simulink model "ringRoad"  (R2018b)
settings: Solver=FixedStepAuto  StartTime=0.0  StopTime=90  FixedStep=0.01  RelTol=1e-3
undefined symbols (not defined in the file or in its folder): Angular, Linear
libraries: robotlib x10, vehdynlibsteering x3, autolibshared x2, autolibutils x2, peGeneralControl x1, dspstat3 x1
settings Model: Creator=ckreienk  LastModifiedBy=ckreienk

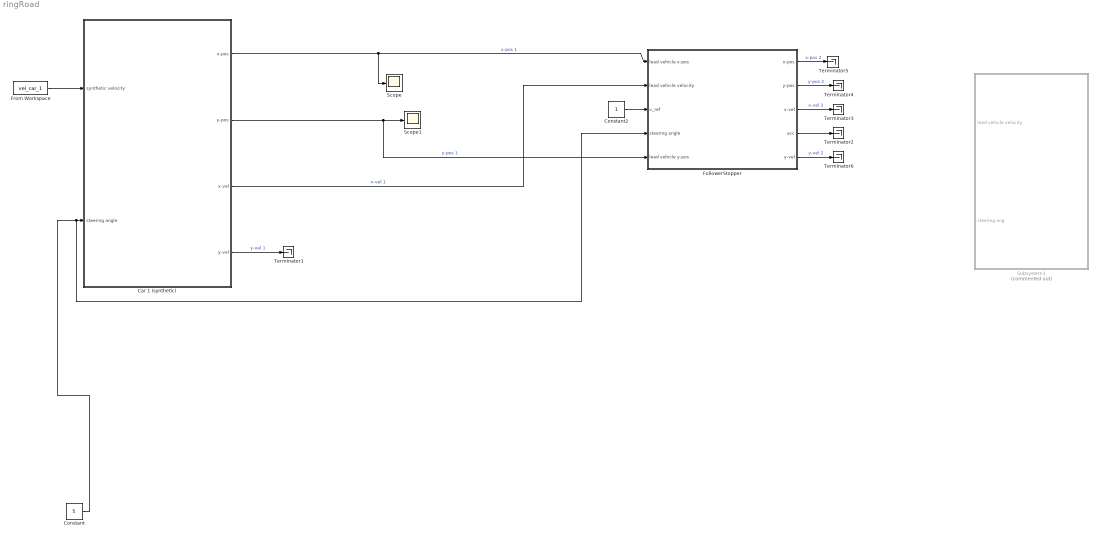
== system ringRoad ==
  Car 1 (synthetic) : Subsystem
  Constant : Constant  Value=5
  Constant2 : Constant
  FollowerStopper : Subsystem
  From Workspace : FromWorkspace  VariableName=vel_car_1
  Scope : Scope
  Scope1 : Scope
  Subsystem1 : Subsystem  Commented=on
  Terminator{1..6} (6 alike) : Terminator
  wires:
  Car 1 (synthetic)/1(x-pos) -> Scope/1, FollowerStopper/1(lead vehicle x-pos)  "x-pos 1"
  Car 1 (synthetic)/3(x-vel) -> FollowerStopper/2(lead vehicle velocity)  "x-vel 1"
  Car 1 (synthetic)/2(y-pos) -> Scope1/1, FollowerStopper/5(lead vehicle y-pos)  "y-pos 1"
  Car 1 (synthetic)/4(y-vel) -> Terminator1/1  "y-vel 1"
  Constant/1 -> FollowerStopper/4(steering angle), Car 1 (synthetic)/2(steering angle)
  From Workspace/1 -> Car 1 (synthetic)/1(synthetic velocity)
  Constant2/1 -> FollowerStopper/3(v_ref)
  FollowerStopper/4(acc) -> Terminator2/1
  FollowerStopper/3(x-vel) -> Terminator3/1  "x-vel 2"
  FollowerStopper/2(y-pos) -> Terminator4/1  "y-pos 2"
  FollowerStopper/1(x-pos) -> Terminator5/1  "x-pos 2"
  FollowerStopper/5(y-vel) -> Terminator6/1  "y-vel 2"

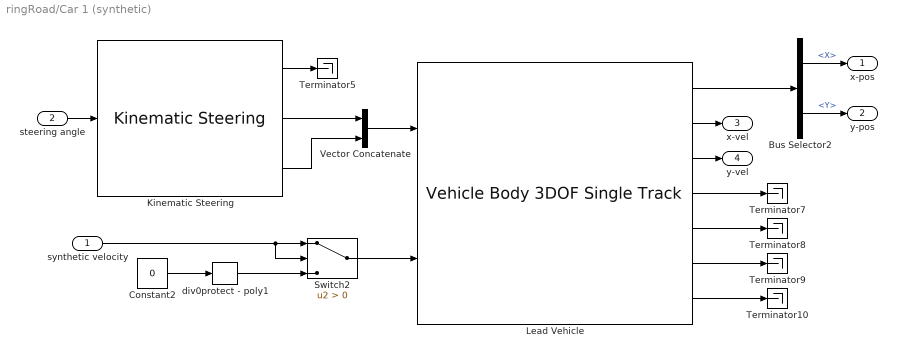
== system ringRoad/Car 1 (synthetic) ==
  synthetic velocity : Inport
  steering angle : Inport  Port=2
  Bus Selector2 : BusSelector  OutputSignals=InertFrm.Geom.Disp.X,InertFrm.Geom.Disp.Y
  Constant2 : Constant  Value=0
  Kinematic Steering : vehdynlibsteering/Kinematic Steering  StrgType=Ackerman  StrgRatioType=Constant  Loc=Front  NrmlFctr=0.01  TrckWdth=1  WhlBase=1.524  Db=0  StrgRng=1.25*pi  StrgAngBpts="[-6.2832   -5.0265   -3.7699   -2.5133   -1.2566         0    1.2566    2.5133    3.7699    5.0265    6.2832]"  StrgRatioTbl=|  StrgRatio=100  StrgArmLngth=0.1  RckCsLngth=0.5  TieRodLngth=0.248  D=0.2  PnnRadius=0.0057  PnnRadiusTbl="[0.0055    0.0055    0.0056    0.0057    0.0058    0.0057    0.0057    0.0057    0.0056    0.0055    0.0055]"  RodLngth=0.1  ParaArmLngth=0.9  aMode=2
      | [13.5000   13.3750   13.2500   13.1250   13.0000   13.0000   13.0000   13.1250   13.2500   13.3750   13.5000
      | ]
      settings: SourceProductName=Vehicle Dynamics Blockset
  Lead Vehicle : autolibshared/Vehicle Body 3DOF Single Track  trackMode=Dual  inputMode=External longitudinal velocity  frontSteerMode=on  rearSteerMode=off  windMode=off  muMode=off  extFMode=off  extMMode=off  aMode=2  NF=2  NR=2  m=2000  a=1.4  b=1.6  h=0.35  X_o=0  xdot_o=0  CalphaMode=off  sigmaMode=on  d=0  w=[1.4,1.4]  Cy_f=12e3  Cy_r=11e3  sigma_f=.1  sigma_r=.1  alpha_f_brk=[-.1 .1]  Cy_f_data=[-9e3 9e3]  alpha_r_brk=[-.1 .1]  Cy_r_data=[-9e3 9e3]  Y_o=0  ydot_o=0  Izz=4000  psi_o=0  r_o=0  Af=2  Cd=.3  Cl=.1  Cpm=.1  beta_w=[0:0.01:0.3]  Cs=[0:0.03:0.9]  Cym=[0:0.01:0.3]  Pabs=101325  Tair=273  g=9.81  mu=1  xdot_tol=.01  Fznom=5000  Fxtire_sat=7e4  Fytire_sat=7e4  longOff=0  latOff=0  vertOff=0
      settings: SourceProductName=Powertrain Blockset  SourceProductBaseCode=PW
  Switch2 : Switch  Criteria=u2 > Threshold
  Terminator{5,7..10} (5 alike) : Terminator
  Vector Concatenate : Concatenate
  div0protect - poly1 : autolibutils/div0protect - poly  thresh=1e-3  aMode=2
      settings: SourceProductName=Powertrain Blockset  SourceProductBaseCode=PW
  x-pos : Outport
  y-pos : Outport  Port=2
  x-vel : Outport  Port=3
  y-vel : Outport  Port=4
  wires:
  Lead Vehicle/6 -> Terminator9/1
  Lead Vehicle/4 -> Terminator7/1
  div0protect - poly1/1 -> Switch2/3
  Lead Vehicle/5 -> Terminator8/1
  Vector Concatenate/1 -> Lead Vehicle/1
  Lead Vehicle/7 -> Terminator10/1
  Kinematic Steering/2 -> Vector Concatenate/1
  Kinematic Steering/1 -> Terminator5/1
  synthetic velocity/1 -> Switch2/2, Switch2/1
  Switch2/1 -> Lead Vehicle/2
  Lead Vehicle/1 -> Bus Selector2/1
  Lead Vehicle/2 -> x-vel/1
  Bus Selector2/1 -> x-pos/1  "<X>"
  Bus Selector2/2 -> y-pos/1  "<Y>"
  Constant2/1 -> div0protect - poly1/1
  steering angle/1 -> Kinematic Steering/1
  Lead Vehicle/3 -> y-vel/1
  Kinematic Steering/3 -> Vector Concatenate/2

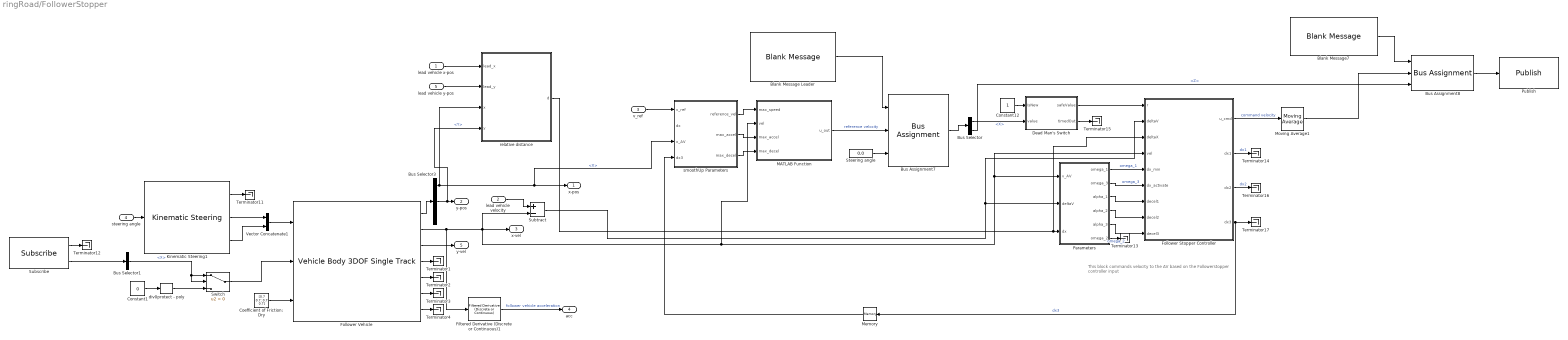
== system ringRoad/FollowerStopper ==
  note: This block commands velocity to the AV based
      | on the Followerstopper controller input
  lead vehicle x-pos : Inport
  lead vehicle velocity : Inport  Port=2
  v_ref : Inport  Port=3
  steering angle : Inport  Port=4
  lead vehicle y-pos : Inport  Port=5
  Blank Message Leader : robotlib/Blank Message  messageClass=Message  entityType=geometry_msgs/Twist  messageType=geometry_msgs/Twist  SampleTime=inf
      settings: SourceProductBaseCode=RO
  Blank Message7 : robotlib/Blank Message  messageClass=Message  entityType=geometry_msgs/Twist  messageType=geometry_msgs/Twist  SampleTime=inf
      settings: SourceProductBaseCode=RO
  Bus Assignment7 : BusAssignment  AssignedSignals=Linear.X,Angular.Z
  Bus Assignment8 : BusAssignment  AssignedSignals=Linear.X,Angular.Z
  Bus Selector : BusSelector  OutputSignals=Linear.X,Angular.Z
  Bus Selector1 : BusSelector  OutputSignals=Linear.X
  Bus Selector3 : BusSelector  OutputSignals=InertFrm.Geom.Disp.X,InertFrm.Geom.Disp.Y,InertFrm.Geom.Disp.Z
  Coefficient of Friction: Dry : Constant  Value=[0.7 0.7; 0.7 0.7]
  Constant1 : Constant  Value=0
  Constant12 : Constant
  Dead Man's Switch : Subsystem  TreatAsAtomicUnit=on  mask{stepSize=0.05, timeout=0.2}
      mask prompts: stepSize "Simulation step size"; timeout "Timeout (in seconds)"
      mask help: Interprets whether a new message has been recently received, and if so permits the data in 'value' to be passed through. Otherwise, 0 is outputted from 'safeValue'
      mask Help: Interprets whether a new message has been recently received, and if so permits the data in 'value' to be passed through. Otherwise, 0 is outputted from 'safeValue'
  Filtered Derivative (Discrete or Continuous)1 : peGeneralControl/Filtered Derivative (Discrete or Continuous)  K=1  T=0.1  B=20  A=-20  minRatio=10  Ts=-1
  Follower Stopper Controller : Subsystem
  Follower Vehicle : autolibshared/Vehicle Body 3DOF Single Track  trackMode=Dual  inputMode=External longitudinal velocity  frontSteerMode=on  rearSteerMode=off  windMode=off  muMode=on  extFMode=off  extMMode=off  aMode=2  NF=2  NR=2  m=2000  a=1.4  b=1.6  h=0.35  X_o=-5.9  xdot_o=0  CalphaMode=off  sigmaMode=on  d=0  w=[1.4,1.4]  Cy_f=12e3  Cy_r=11e3  sigma_f=.1  sigma_r=.1  alpha_f_brk=[-.1 .1]  Cy_f_data=[-9e3 9e3]  alpha_r_brk=[-.1 .1]  Cy_r_data=[-9e3 9e3]  Y_o=0.3  ydot_o=0  Izz=4000  psi_o=0  r_o=0  Af=2  Cd=.3  Cl=.1  Cpm=.1  beta_w=[0:0.01:0.3]  Cs=[0:0.03:0.9]  Cym=[0:0.01:0.3]  Pabs=101325  Tair=273  g=9.81  mu=1  xdot_tol=.01  Fznom=5000  Fxtire_sat=7e4  Fytire_sat=7e4  longOff=0  latOff=0  vertOff=0
      settings: SourceProductName=Powertrain Blockset  SourceProductBaseCode=PW
  Kinematic Steering1 : vehdynlibsteering/Kinematic Steering  StrgType=Ackerman  StrgRatioType=Constant  Loc=Front  NrmlFctr=0.01  TrckWdth=1  WhlBase=1.524  Db=0  StrgRng=1.25*pi  StrgAngBpts="[-6.2832   -5.0265   -3.7699   -2.5133   -1.2566         0    1.2566    2.5133    3.7699    5.0265    6.2832]"  StrgRatioTbl=|  StrgRatio=100  StrgArmLngth=0.1  RckCsLngth=0.5  TieRodLngth=0.248  D=0.2  PnnRadius=0.0057  PnnRadiusTbl="[0.0055    0.0055    0.0056    0.0057    0.0058    0.0057    0.0057    0.0057    0.0056    0.0055    0.0055]"  RodLngth=0.1  ParaArmLngth=0.9  aMode=2
      | [13.5000   13.3750   13.2500   13.1250   13.0000   13.0000   13.0000   13.1250   13.2500   13.3750   13.5000
      | ]
      settings: SourceProductName=Vehicle Dynamics Blockset
  MATLAB Function : MATLAB Function  TreatAsAtomicUnit=on
  Memory : Memory  InheritSampleTime=on
  Moving Average1 : dspstat3/Moving Average  Method=Sliding window  ForgettingFactorPort=off  SpecifyWindowLength=on  WindowLength=10  ForgettingFactor=0.9  SimulateUsing=Code generation
  Parameters : Subsystem
  Publish : robotlib/Publish  topicSource=Specify your own  topic=cmd_vel  messageType=geometry_msgs/Twist  messageQueueLength=1
      settings: SourceProductBaseCode=RO
  Steering angle : Constant  Value=0.0
  Subscribe : robotlib/Subscribe  topicSource=Specify your own  topic=cmd_vel  messageType=geometry_msgs/Twist  sampleTime=-1  messageQueueLength=1
      settings: SourceProductBaseCode=RO
  Subtract : Sum  Inputs=+-
  Switch : Switch  Criteria=u2 > Threshold
  Terminator{1..4,11..17} (11 alike) : Terminator
  Vector Concatenate1 : Concatenate
  div0protect - poly : autolibutils/div0protect - poly  thresh=1e-3  aMode=2
      settings: SourceProductName=Powertrain Blockset  SourceProductBaseCode=PW
  relative distance : MATLAB Function  TreatAsAtomicUnit=on
  smoothUp Parameters : Subsystem
  x-pos : Outport
  y-pos : Outport  Port=2
  x-vel : Outport  Port=3
  acc : Outport  Port=4
  y-vel : Outport  Port=5
  wires:
  Dead Man's Switch/2(timedOut) -> Terminator15/1
  Bus Selector/2 -> Bus Assignment8/3  "<Z>"
  Vector Concatenate1/1 -> Follower Vehicle/1
  Subscribe/2 -> Bus Selector1/1
  Parameters/5(alpha_3) -> Follower Stopper Controller/9(decel3)
  Parameters/3(alpha_1) -> Follower Stopper Controller/7(decel1)
  Steering angle/1 -> Bus Assignment7/3
  Follower Vehicle/3 -> y-vel/1
  Bus Selector3/1 -> x-pos/1, smoothUp Parameters/3(x_AV), relative distance/3(x)  "<X>"
  Coefficient of Friction: Dry/1 -> Follower Vehicle/3
  div0protect - poly/1 -> Switch/3
  Moving Average1/1 -> Bus Assignment8/2
  Parameters/2(omega_3) -> Follower Stopper Controller/6(dx_activate)  "omega_3"
  lead vehicle velocity/1 -> Subtract/1
  Subscribe/1 -> Terminator12/1
  Follower Vehicle/5 -> Terminator2/1
  Switch/1 -> Follower Vehicle/2
  Constant1/1 -> div0protect - poly/1
  Constant12/1 -> Dead Man's Switch/1(IsNew)
  Bus Selector3/2 -> relative distance/4(y), y-pos/1  "<Y>"
  Parameters/4(alpha_2) -> Follower Stopper Controller/8(decel2)
  Follower Vehicle/2 -> Filtered Derivative (Discrete or Continuous)1/1, Follower Stopper Controller/4(vel), Parameters/1(v_AV), MATLAB Function/2(vel), x-vel/1, Subtract/2
  Parameters/6(omega_2) -> Terminator13/1  "omega_2"
  Follower Vehicle/4 -> Terminator1/1
  Follower Stopper Controller/3(dx2) -> Terminator16/1  "dx2"
  Follower Stopper Controller/2(dx1) -> Terminator14/1  "dx1"
  Follower Vehicle/1 -> Bus Selector3/1
  Bus Selector1/1 -> Switch/1, Switch/2  "<X>"
  smoothUp Parameters/2(max_accel) -> MATLAB Function/3(max_accel)
  Blank Message Leader/1 -> Bus Assignment7/1
  Kinematic Steering1/2 -> Vector Concatenate1/1
  Dead Man's Switch/1(safeValue) -> Follower Stopper Controller/1(r)
  Bus Assignment8/1 -> Publish/1
  Follower Stopper Controller/4(dx3) -> Memory/1, Terminator17/1  "dx3"
  Kinematic Steering1/3 -> Vector Concatenate1/2
  Bus Selector/1 -> Dead Man's Switch/2(value)  "<X>"
  Follower Vehicle/7 -> Terminator4/1
  v_ref/1 -> smoothUp Parameters/1(v_ref)
  Kinematic Steering1/1 -> Terminator11/1
  smoothUp Parameters/1(reference_vel) -> MATLAB Function/1(max_speed)
  smoothUp Parameters/3(max_decel) -> MATLAB Function/4(max_decel)
  steering angle/1 -> Kinematic Steering1/1
  Bus Assignment7/1 -> Bus Selector/1
  Filtered Derivative (Discrete or Continuous)1/1 -> acc/1  "follower vehicle acceleration"
  Parameters/1(omega_1) -> Follower Stopper Controller/5(dx_min)  "omega_1"
  Follower Stopper Controller/1(u_cmd) -> Moving Average1/1  "command velocity"
  MATLAB Function/1(u_out) -> Bus Assignment7/2  "reference velocity"
  Blank Message7/1 -> Bus Assignment8/1
  Subtract/1 -> Follower Stopper Controller/2(deltaV), Parameters/2(deltaV)
  Memory/1 -> smoothUp Parameters/4(dx3)
  Follower Vehicle/6 -> Terminator3/1
  lead vehicle x-pos/1 -> relative distance/1(lead_x)
  lead vehicle y-pos/1 -> relative distance/2(lead_y)
  relative distance/1(d) -> Follower Stopper Controller/3(deltaX), Parameters/3(dx)

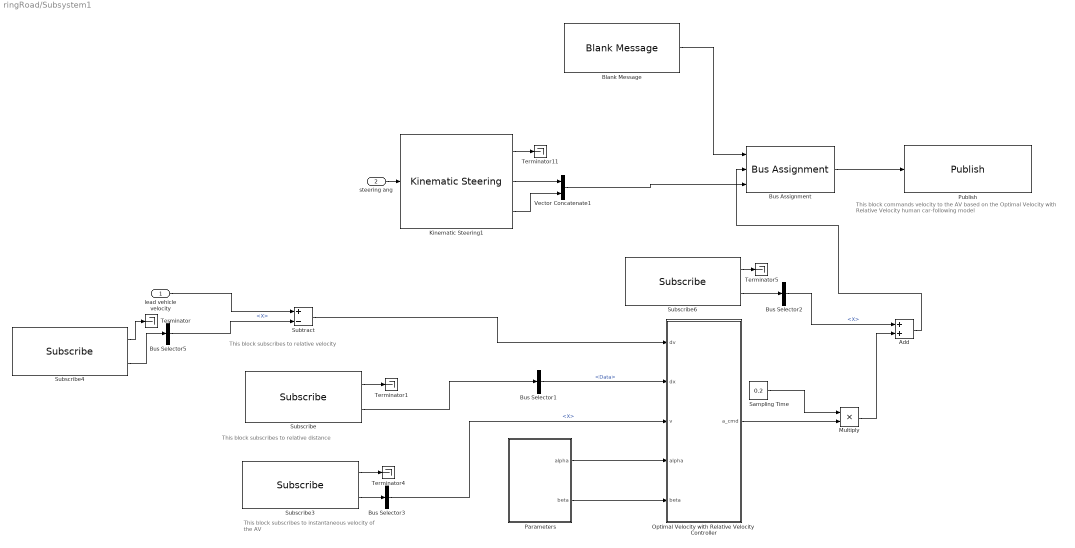
== system ringRoad/Subsystem1 ==
  note: This block subscribes to relative velocity
  note: This block subscribes to relative distance
  note: This block subscribes to
      | instantaneous velocity of the AV
  note: This block commands velocity to the AV based
      | on the Optimal Velocity with Relative Velocity
      | human car-following model
  lead vehicle velocity : Inport
  steering ang : Inport  Port=2
  Add : Sum
  Blank Message : robotlib/Blank Message  messageClass=Message  entityType=geometry_msgs/Twist  messageType=geometry_msgs/Twist  SampleTime=inf
      settings: SourceProductBaseCode=RO
  Bus Assignment : BusAssignment  AssignedSignals=Linear.X,Angular.Z
  Bus Selector1 : BusSelector  OutputSignals=Data
  Bus Selector2 : BusSelector  OutputSignals=Linear.X
  Bus Selector3 : BusSelector  OutputSignals=Linear.X
  Bus Selector5 : BusSelector  OutputSignals=Linear.X
  Kinematic Steering1 : vehdynlibsteering/Kinematic Steering  StrgType=Ackerman  StrgRatioType=Constant  Loc=Front  NrmlFctr=0.01  TrckWdth=1  WhlBase=1.524  Db=0  StrgRng=1.25*pi  StrgAngBpts="[-6.2832   -5.0265   -3.7699   -2.5133   -1.2566         0    1.2566    2.5133    3.7699    5.0265    6.2832]"  StrgRatioTbl=|  StrgRatio=100  StrgArmLngth=0.1  RckCsLngth=0.5  TieRodLngth=0.248  D=0.2  PnnRadius=0.0057  PnnRadiusTbl="[0.0055    0.0055    0.0056    0.0057    0.0058    0.0057    0.0057    0.0057    0.0056    0.0055    0.0055]"  RodLngth=0.1  ParaArmLngth=0.9  aMode=2
      | [13.5000   13.3750   13.2500   13.1250   13.0000   13.0000   13.0000   13.1250   13.2500   13.3750   13.5000
      | ]
      settings: SourceProductName=Vehicle Dynamics Blockset
  Multiply : Product
  Optimal Velocity with Relative Velocity Controller : Subsystem
  Parameters : Subsystem
  Publish : robotlib/Publish  topicSource=Select from ROS network  topic=/followerVehicle/cmd_vel  messageType=geometry_msgs/Twist  messageQueueLength=1
      settings: SourceProductBaseCode=RO
  Sampling Time : Constant  Value=0.2
  Subscribe : robotlib/Subscribe  topicSource=Select from ROS network  topic=/followerVehicle/distanceEstimatorSteeringBased/dist  messageType=std_msgs/Float64  sampleTime=-1  messageQueueLength=1
      settings: SourceProductBaseCode=RO
  Subscribe3 : robotlib/Subscribe  topicSource=Select from ROS network  topic=/followerVehicle/cmd_vel  messageType=geometry_msgs/Twist  sampleTime=-1  messageQueueLength=1
      settings: SourceProductBaseCode=RO
  Subscribe4 : robotlib/Subscribe  topicSource=Select from ROS network  topic=/followerVehicle/cmd_vel  messageType=geometry_msgs/Twist  sampleTime=-1  messageQueueLength=1
      settings: SourceProductBaseCode=RO
  Subscribe6 : robotlib/Subscribe  topicSource=Select from ROS network  topic=/followerVehicle/cmd_vel  messageType=geometry_msgs/Twist  sampleTime=-1  messageQueueLength=1
      settings: SourceProductBaseCode=RO
  Subtract : Sum  Inputs=+-
  Terminator{,1,4..5,11} (5 alike) : Terminator
  Vector Concatenate1 : Concatenate
  wires:
  Sampling Time/1 -> Multiply/1
  Multiply/1 -> Add/2
  Optimal Velocity with Relative Velocity Controller/1(a_cmd) -> Multiply/2
  Parameters/1(alpha) -> Optimal Velocity with Relative Velocity Controller/4(alpha)
  Bus Selector3/1 -> Optimal Velocity with Relative Velocity Controller/3(v)  "<X>"
  lead vehicle velocity/1 -> Subtract/1
  Bus Selector1/1 -> Optimal Velocity with Relative Velocity Controller/2(dx)  "<Data>"
  Subscribe3/2 -> Bus Selector3/1
  Subscribe/1 -> Terminator1/1
  Parameters/2(beta) -> Optimal Velocity with Relative Velocity Controller/5(beta)
  Subscribe3/1 -> Terminator4/1
  Bus Selector2/1 -> Add/1  "<X>"
  Add/1 -> Bus Assignment/2
  Subscribe4/2 -> Bus Selector5/1
  Subscribe4/1 -> Terminator/1
  Subscribe6/2 -> Bus Selector2/1
  Subscribe/2 -> Bus Selector1/1
  Blank Message/1 -> Bus Assignment/1
  Subtract/1 -> Optimal Velocity with Relative Velocity Controller/1(dv)
  Bus Assignment/1 -> Publish/1
  Bus Selector5/1 -> Subtract/2  "<X>"
  Subscribe6/1 -> Terminator5/1
  Kinematic Steering1/1 -> Terminator11/1
  Vector Concatenate1/1 -> Bus Assignment/3
  Kinematic Steering1/3 -> Vector Concatenate1/2
  Kinematic Steering1/2 -> Vector Concatenate1/1
  steering ang/1 -> Kinematic Steering1/1

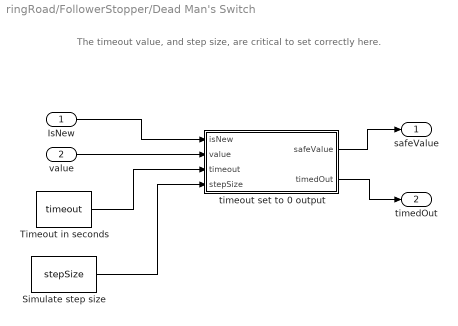
== system ringRoad/FollowerStopper/Dead Man's Switch ==
  note: The timeout value, and step size, are critical to set correctly here.
  IsNew : Inport
  value : Inport  Port=2
  Simulate step size : Constant  Value=stepSize
  Timeout in seconds : Constant  Value=timeout
  timeout set to 0 output : MATLAB Function  TreatAsAtomicUnit=on
  safeValue : Outport  InitialOutput=[0]
  timedOut : Outport  Port=2  InitialOutput=[0]
  wires:
  Simulate step size/1 -> timeout set to 0 output/4(stepSize)
  timeout set to 0 output/2(timedOut) -> timedOut/1
  Timeout in seconds/1 -> timeout set to 0 output/3(timeout)
  value/1 -> timeout set to 0 output/2(value)
  timeout set to 0 output/1(safeValue) -> safeValue/1
  IsNew/1 -> timeout set to 0 output/1(isNew)

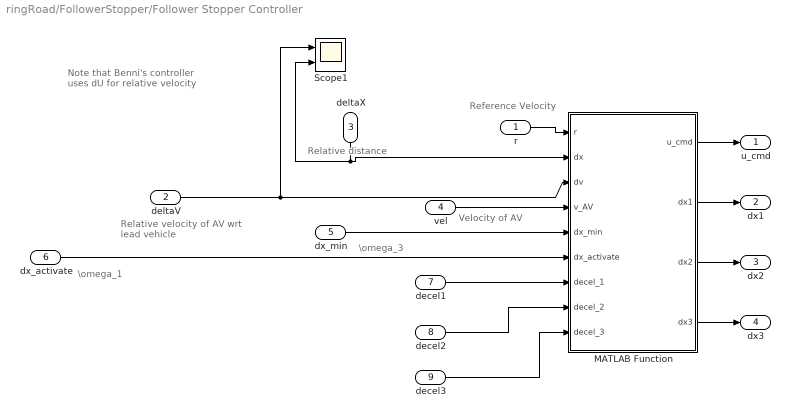
== system ringRoad/FollowerStopper/Follower Stopper Controller ==
  note: \omega_3
  note: \omega_1
  note: Relative distance
  note: Reference Velocity
  note: Velocity of AV
  note: Relative velocity of
      | AV wrt lead vehicle
  note: Note that Benni's
      | controller uses dU
      | for relative
      | velocity
  r : Inport
  deltaV : Inport  Port=2
  deltaX : Inport  Port=3
  vel : Inport  Port=4
  dx_min : Inport  Port=5
  dx_activate : Inport  Port=6
  decel1 : Inport  Port=7
  decel2 : Inport  Port=8
  decel3 : Inport  Port=9
  MATLAB Function : MATLAB Function  TreatAsAtomicUnit=on
  Scope1 : Scope  NumInputPorts=2
  u_cmd : Outport
  dx1 : Outport  Port=2
  dx2 : Outport  Port=3
  dx3 : Outport  Port=4
  wires:
  r/1 -> MATLAB Function/1(r)
  dx_activate/1 -> MATLAB Function/6(dx_activate)
  dx_min/1 -> MATLAB Function/5(dx_min)
  vel/1 -> MATLAB Function/4(v_AV)
  MATLAB Function/1(u_cmd) -> u_cmd/1
  deltaV/1 -> Scope1/1, MATLAB Function/3(dv)
  deltaX/1 -> Scope1/2, MATLAB Function/2(dx)
  decel3/1 -> MATLAB Function/9(decel_3)
  decel2/1 -> MATLAB Function/8(decel_2)
  decel1/1 -> MATLAB Function/7(decel_1)
  MATLAB Function/2(dx1) -> dx1/1
  MATLAB Function/3(dx2) -> dx2/1
  MATLAB Function/4(dx3) -> dx3/1

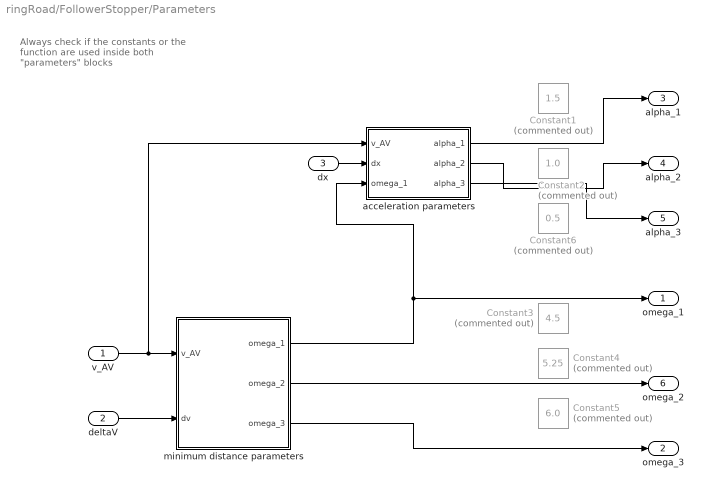
== system ringRoad/FollowerStopper/Parameters ==
  note: Always check if the constants or the function are used inside both "parameters" blocks
  v_AV : Inport
  deltaV : Inport  Port=2
  dx : Inport  Port=3
  Constant1 : Constant  Commented=on  Value=1.5
  Constant2 : Constant  Commented=on  Value=1.0
  Constant3 : Constant  Commented=on  Value=4.5
  Constant4 : Constant  Commented=on  Value=5.25
  Constant5 : Constant  Commented=on  Value=6.0
  Constant6 : Constant  Commented=on  Value=0.5
  acceleration parameters : MATLAB Function  TreatAsAtomicUnit=on
  minimum distance parameters : MATLAB Function  TreatAsAtomicUnit=on
  omega_1 : Outport
  omega_3 : Outport  Port=2
  alpha_1 : Outport  Port=3
  alpha_2 : Outport  Port=4
  alpha_3 : Outport  Port=5
  omega_2 : Outport  Port=6
  wires:
  deltaV/1 -> minimum distance parameters/2(dv)
  dx/1 -> acceleration parameters/2(dx)
  v_AV/1 -> acceleration parameters/1(v_AV), minimum distance parameters/1(v_AV)
  minimum distance parameters/1(omega_1) -> omega_1/1, acceleration parameters/3(omega_1)
  minimum distance parameters/2(omega_2) -> omega_2/1
  minimum distance parameters/3(omega_3) -> omega_3/1
  acceleration parameters/1(alpha_1) -> alpha_1/1
  acceleration parameters/2(alpha_2) -> alpha_2/1
  acceleration parameters/3(alpha_3) -> alpha_3/1

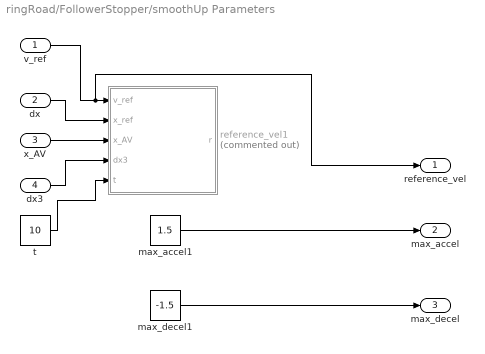
== system ringRoad/FollowerStopper/smoothUp Parameters ==
  v_ref : Inport
  dx : Inport  Port=2
  x_AV : Inport  Port=3
  dx3 : Inport  Port=4
  max_accel1 : Constant  Value=1.5
  max_decel1 : Constant  Value=-1.5
  reference_vel1 : MATLAB Function  Commented=on  TreatAsAtomicUnit=on
  t : Constant  Value=10
  reference_vel : Outport
  max_accel : Outport  Port=2
  max_decel : Outport  Port=3
  wires:
  max_accel1/1 -> max_accel/1
  max_decel1/1 -> max_decel/1
  v_ref/1 -> reference_vel/1, reference_vel1/1(v_ref)
  dx3/1 -> reference_vel1/4(dx3)
  x_AV/1 -> reference_vel1/3(x_AV)
  dx/1 -> reference_vel1/2(x_ref)
  t/1 -> reference_vel1/5(t)

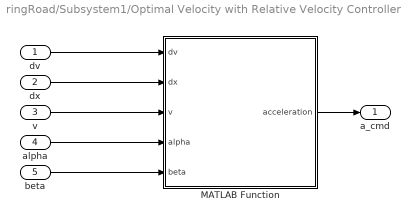
== system ringRoad/Subsystem1/Optimal Velocity with Relative Velocity Controller ==
  dv : Inport
  dx : Inport  Port=2
  v : Inport  Port=3
  alpha : Inport  Port=4
  beta : Inport  Port=5
  MATLAB Function : MATLAB Function  TreatAsAtomicUnit=on
  a_cmd : Outport
  wires:
  MATLAB Function/1(acceleration) -> a_cmd/1
  v/1 -> MATLAB Function/3(v)
  alpha/1 -> MATLAB Function/4(alpha)
  beta/1 -> MATLAB Function/5(beta)
  dv/1 -> MATLAB Function/1(dv)
  dx/1 -> MATLAB Function/2(dx)

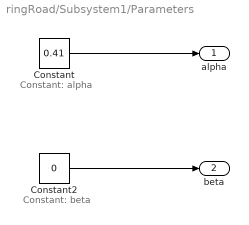
== system ringRoad/Subsystem1/Parameters ==
  note: Constant: beta
  note: Constant: alpha
  Constant : Constant  Value=0.41
  Constant2 : Constant  Value=0
  alpha : Outport
  beta : Outport  Port=2
  wires:
  Constant/1 -> alpha/1
  Constant2/1 -> beta/1

== matlab function ringRoad/FollowerStopper/Dead Man's Switch/timeout set to 0 output ==
  data: isNew input; safeValue output; value input; timeout input; timedOut output; stepSize input
function [safeValue,timedOut] = fcn(isNew,value,timeout,stepSize)
%#codegen
persistent sinceLastMsg
timedOut=true;
if isempty(sinceLastMsg)
    sinceLastMsg=(timeout/stepSize)+1;
end

safeValue=0;
% if no new message
% after timeout, we output 0
if( isNew == true )
    sinceLastMsg = 0;
else
    sinceLastMsg = sinceLastMsg+1;
end

% Note: we require step size as an input here, and depend on our
% system being executed at a regular rate, or bad things will happen
if( sinceLastMsg < timeout/stepSize )
    timedOut = false;
end
    
if( timedOut == false )
    safeValue = value;
end

== matlab function ringRoad/FollowerStopper/MATLAB Function ==
  settings: updateMethod=DISCRETE
  data: max_speed input; u_out output; vel input; max_accel input; max_decel input
function u_out = fcn(max_speed,vel,max_accel,max_decel)
% #codegen
persistent y

if isempty(y)
    y=vel;
end

dt=0.01;
if( y > max_speed + max_accel*dt)
    y = max(max_speed,y - abs(max_decel)*dt);
elseif( y < max_speed - abs(max_decel)*dt)
    y = min(max_speed,y + max_accel*dt);
else
    y = max_speed;
end

u_out = y;

== matlab function ringRoad/Subsystem1/Optimal Velocity with Relative Velocity Controller/MATLAB Function ==
  data: dv input; dx input; v input; alpha input; acceleration output; beta input
function acceleration = fcn(dv, dx, v, alpha, beta)
eqSpeedSpacing = tanh(dx-2)+tanh(2);
acceleration = alpha*(eqSpeedSpacing - v) + beta*dv

== matlab function ringRoad/FollowerStopper/Parameters/acceleration parameters ==
  data: v_AV input; alpha_1 output; dx input; omega_1 input; alpha_2 output; alpha_3 output
function [alpha_1,alpha_2,alpha_3] = fcn(v_AV,dx,omega_1)

% alpha_2 = 0.15*9.80665;
% alpha_1 = max(v_AV^2/(2*(dx-omega_1)),alpha_2);
% alpha_3 = alpha_2-(alpha_1-alpha_2);

alpha_1 = 1.5;
alpha_2 = 1.0;
alpha_3 = 0.5;

== matlab function ringRoad/FollowerStopper/Parameters/minimum distance parameters ==
  data: v_AV input; omega_1 output; dv input; omega_2 output; omega_3 output
function [omega_1, omega_2, omega_3] = fcn(v_AV,dv)

% v_lead = max(v_AV + dv,0);
% omega_1 = 1;
% omega_2 = max(omega_1,2.766*v_AV);
% omega_3 = (omega_2-omega_1) + omega_2;

omega_1 = 4.5;
omega_2 = 5.25;
omega_3 = 6.0;

== matlab function ringRoad/FollowerStopper/Follower Stopper Controller/MATLAB Function ==
  data: r input; u_cmd output; dx input; dv input; v_AV input; dx_min input; dx_activate input; decel_1 input; decel_2 input; decel_3 input; dx1 output; dx2 output; dx3 output
function [u_cmd,dx1,dx2,dx3] = fcn(r,dx,dv,v_AV,...
    dx_min,dx_activate,decel_1,decel_2,decel_3)
%#codegen
% Safety controller, based on quadratic bands.
% Input: r = desired velocity (from other models)
%          dx = estimate of gap to vehicle ahead
%          dv = estimate of time derivative of dx (= velocity difference)
%         v_AV = velocity of AV
%      dx_min = minimum distance
% dx_activate = distance below which controller does something
%       decel = vector of three deceleration values for parabolas
% Out:  u_cmd = actual velocity commanded (always u_cmd<=U)
%
% Controller-specific parameters
dx_mid = (dx_min+dx_activate)/2; % mid distance, where v_lead is commanded
% Lead vehicle velocity
v_lead = v_AV+dv; % velocity of lead vehicle
v_lead = max(v_lead,0); % lead vehicle cannot go backwards
v = min(r,v_lead); % safety velocity cannot exceed desired velocity U
% Treatment of positive dv-values
dv = min(dv,0); % domains for dv>0 same as dv=0
% For given dv, dx-values of band boundaries
dx1 = dx_min+1/(2*decel_1)*dv.^2;
dx2 = dx_mid+1/(2*decel_2)*dv.^2;
dx3 = dx_activate+1/(2*decel_3)*dv.^2;

% Actual commanded velocity
dt = 0.01;
max_accel = 1.5;
smoothChange = v_AV + max_accel*dt;
if (dx <= dx1)
    u_cmd = 0;
elseif (dx <= dx2)
    u_cmd = min(v*(dx-dx1)/(dx2-dx1) , smoothChange);
elseif (dx <= dx3)
    u_cmd = min(v + (r-v)*(dx-dx2)/(dx3-dx2) , smoothChange);
else
    u_cmd = min(r , smoothChange);
end

== matlab function ringRoad/FollowerStopper/smoothUp Parameters/reference_vel1 ==
  data: v_ref input; r output; x_ref input; x_AV input; dx3 input; t input
function r = fcn(v_ref,x_ref,x_AV,dx3,t)

v_ref = max(v_ref,0);
r = v_ref+1/t*((x_ref-x_AV)-dx3);

== matlab function ringRoad/FollowerStopper/relative distance ==
  data: lead_x input; d output; lead_y input; x input; y input
function d = fcn(lead_x,lead_y,x,y)

dx = lead_x-x;
dy = lead_y-y;
d = sqrt(dx^2+dy^2);
